simulink model "PID_Seriell"  (R2024a)
settings: Solver=ode45  StartTime=0.0  StopTime=1  FixedStep=1e-2  RelTol=1e-4  AbsTol=1e-4
values from neighbouring files (symbols this model uses):
  Kp = 9.8    [ITAE_Plots_PT2_limitations Rechenbeispiel.m]
  Td = 0.01    [ITAE_Plots_PT2_limitations Rechenbeispiel.m]
  Ti = 0.11    [ITAE_Plots_PT2_limitations Rechenbeispiel.m]
settings Model: Creator=bhir  LastModifiedBy=Flo
settings SolverCC: AlgebraicLoopSolver=TrustRegion
settings DataIOCC: ReturnWorkspaceOutputs=off
settings DebuggingCC: UnconnectedInputMsg=warning  UnconnectedOutputMsg=warning  UnconnectedLineMsg=warning  ArithmeticOperatorsInVariantConditions=warning
settings SFSimCC: SimUseLocalCustomCode=off  CustomCodeUndefinedFunction=UseInterfaceOnly
settings RTWCC: RTWUseLocalCustomCode=off  GPUComputeCapability=3.5  DLArmComputeVersion=19.05
settings CodeAppCC: StateflowObjectComments=on

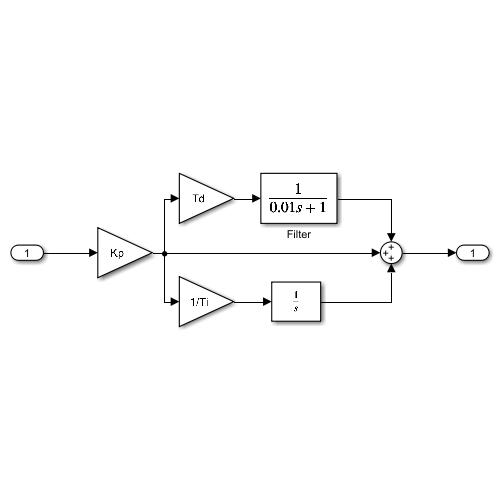
[thumbnail: Simulink's stored preview of the top-level diagram]
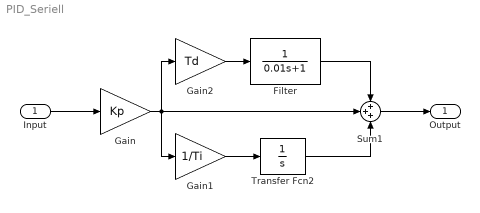
== system PID_Seriell ==
  Input : Inport
  Filter : TransferFcn  Denominator=[0.01 1]
  Gain : Gain  Gain=Kp
  Gain1 : Gain  Gain=1/Ti
  Gain2 : Gain  Gain=Td
  Sum1 : Sum  Inputs=+++
  Transfer Fcn2 : TransferFcn  Denominator=[1 0]
  Output : Outport
  wires:
  Input/1 -> Gain/1
  Gain1/1 -> Transfer Fcn2/1
  Gain/1 -> Gain2/1, Sum1/2, Gain1/1
  Filter/1 -> Sum1/1
  Gain2/1 -> Filter/1
  Sum1/1 -> Output/1
  Transfer Fcn2/1 -> Sum1/3
